simulink model "Controladores"  (R2024b)
settings: Solver=VariableStepAuto  StartTime=0.0  StopTime=10.0  RelTol=1e-3
undefined symbols (not defined in the file or in its folder): qpr, qr
settings Model: Creator=javier  LastModifiedBy=javier

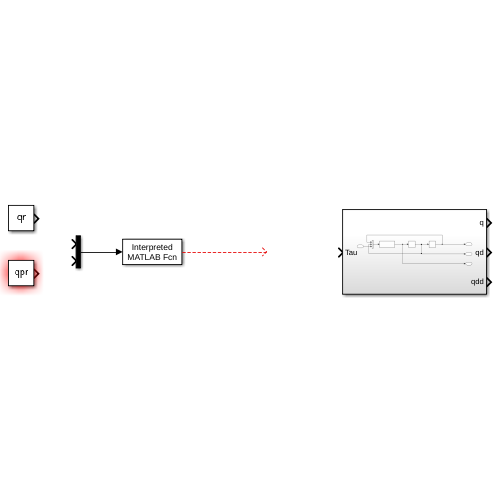
[thumbnail: Simulink's stored preview of the top-level diagram]
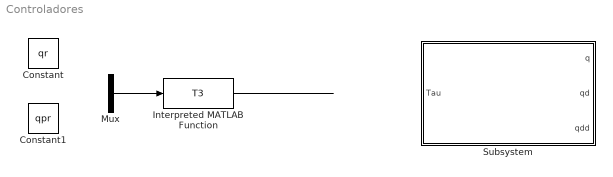
== system Controladores ==
  Constant : Constant  Value=qr
  Constant1 : Constant  Value=qpr
  Interpreted MATLAB Function : MATLABFcn  MATLABFcn=T3  OutputDimensions=2
  Mux : Mux  Inputs=2
  Subsystem : Subsystem
  wires:
  Interpreted MATLAB Function/1 -> ?
  Mux/1 -> Interpreted MATLAB Function/1

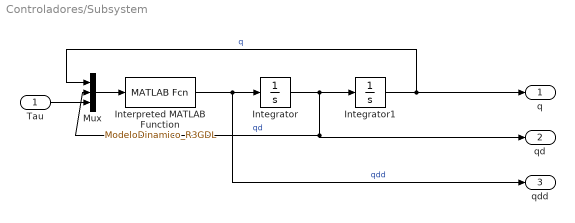
== system Controladores/Subsystem ==
  Tau : Inport
  Integrator : Integrator
  Integrator1 : Integrator
  Interpreted MATLAB Function : MATLABFcn  MATLABFcn=ModeloDinamico_R3GDL  OutputDimensions=3
  Mux : Mux  Inputs=3
  q : Outport
  qd : Outport  Port=2
  qdd : Outport  Port=3
  wires:
  Mux/1 -> Interpreted MATLAB Function/1
  Integrator/1 -> Mux/2, qd/1, Integrator1/1  "qd"
  Interpreted MATLAB Function/1 -> qdd/1, Integrator/1  "qdd"
  Integrator1/1 -> q/1, Mux/1  "q"
  Tau/1 -> Mux/3
